simulink model "discreteSSmodel"  (R2016b)
settings: Solver=FixedStepDiscrete  StartTime=0.0  StopTime=100  FixedStep=0.05  RelTol=1e-3
values from neighbouring files (symbols this model uses):
  Ad = d_sys.A    [ControllerLQR.m]    (also in plotData.m)
  Bd = d_sys.B    [ControllerLQR.m]    (also in plotData.m)
  Cd = d_sys.C    [ControllerLQR.m]    (also in plotData.m)
  F = Fe(1:2,1:3)    [ControllerLQR.m]    (also in robustModel.m = info.KFI(1:2,1:3))
  Ts = 0.05    [ControllerLQR.m]    (also in plotData.m)
undefined symbols (not defined in the file or in its folder): DiscIntNeverNeededParam, Fi
settings Model: Creator=himalkooverjee  LastModifiedBy=himalkooverjee

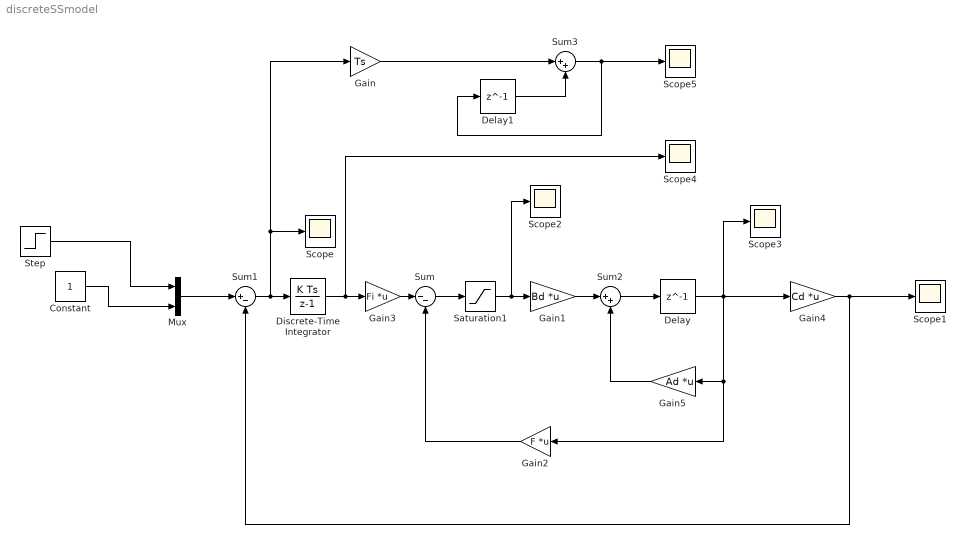
== system discreteSSmodel ==
  Constant : Constant
  Delay : Delay  DelayLength=1
  Delay1 : Delay  DelayLength=1
  Discrete-Time Integrator : DiscreteIntegrator  InitialConditionSetting=State (most efficient)  SampleTime=-1  ICPrevOutput=DiscIntNeverNeededParam  ICPrevScaledInput=DiscIntNeverNeededParam
  Gain : Gain  Gain=Ts
  Gain1 : Gain  Gain=Bd  Multiplication=Matrix(K*u)
  Gain2 : Gain  Gain=F  Multiplication=Matrix(K*u)
  Gain3 : Gain  Gain=Fi  Multiplication=Matrix(K*u)
  Gain4 : Gain  Gain=Cd  Multiplication=Matrix(K*u)
  Gain5 : Gain  Gain=Ad  Multiplication=Matrix(K*u)
  Mux : Mux  Inputs=2
  Saturation1 : Saturate  UpperLimit=40  LowerLimit=0
  Scope{,1..5} (6 alike) : Scope
  Step : Step  Time=50  SampleTime=0
  Sum : Sum  Inputs=|--
  Sum1 : Sum  Inputs=|+-
  Sum2 : Sum  Inputs=|++
  Sum3 : Sum  Inputs=|++
  wires:
  Gain3/1 -> Sum/1
  Sum1/1 -> Gain/1, Scope/1, Discrete-Time Integrator/1
  Discrete-Time Integrator/1 -> Scope4/1, Gain3/1
  Gain2/1 -> Sum/2
  Delay/1 -> Scope3/1, Gain2/1, Gain5/1, Gain4/1
  Mux/1 -> Sum1/1
  Gain4/1 -> Scope1/1, Sum1/2
  Gain1/1 -> Sum2/1
  Gain5/1 -> Sum2/2
  Sum2/1 -> Delay/1
  Saturation1/1 -> Scope2/1, Gain1/1
  Sum/1 -> Saturation1/1
  Sum3/1 -> Delay1/1, Scope5/1
  Delay1/1 -> Sum3/2
  Gain/1 -> Sum3/1
  Step/1 -> Mux/1
  Constant/1 -> Mux/2
